simulink model "lab3_real_integrator"  (R2015a)
settings: Solver=ode3  StartTime=0.0  StopTime=30  RelTol=1e-3
values from neighbouring files (symbols this model uses):
  Ke = -4.2046    [controller_design.m]    (also in controller_test.m)
  Kp = 34.0683    [controller_design.m]    (also in controller_test.m)
  Nbar = Nu+K*Nx    [controller_design.m]    (also in controller_test.m)
  sampling_time = 1/50    (= 0.02)    [controller_design.m]    (also in controller_test.m)
undefined symbols (not defined in the file or in its folder): A, B, C, K, M, MIO, National_Instruments, PCI
libraries: sldrtlib x2
settings Model: SimulationMode=external  ExtModeTrigDuration=200000  Creator=alunos  LastModifiedBy=alunos
settings DataIOCC: LimitDataPoints=off
settings HardwareCC: ProdBitPerPointer=64  ProdLargestAtomicFloat=Float  ProdIntDivRoundTo=Zero  ProdEndianess=LittleEndian  ProdHWDeviceType=Specified  TargetIntDivRoundTo=Zero  TargetEndianess=LittleEndian  TargetHWDeviceType=Intel->x86/Pentium
settings RTWCC: SystemTargetFile=rtwin.tlc  TemplateMakefile=rtwin.tmf  Description=Simulink Desktop Real-Time  RTWCompilerOptimization=on
settings CodeAppCC: MaxIdLength=95
settings RTWinTargetCC: TargetPreCompLibLocation=C:\Program Files\MATLAB\R2017a\toolbox\sldrt\lib\win64  ExtModeMexFile=sldrtext

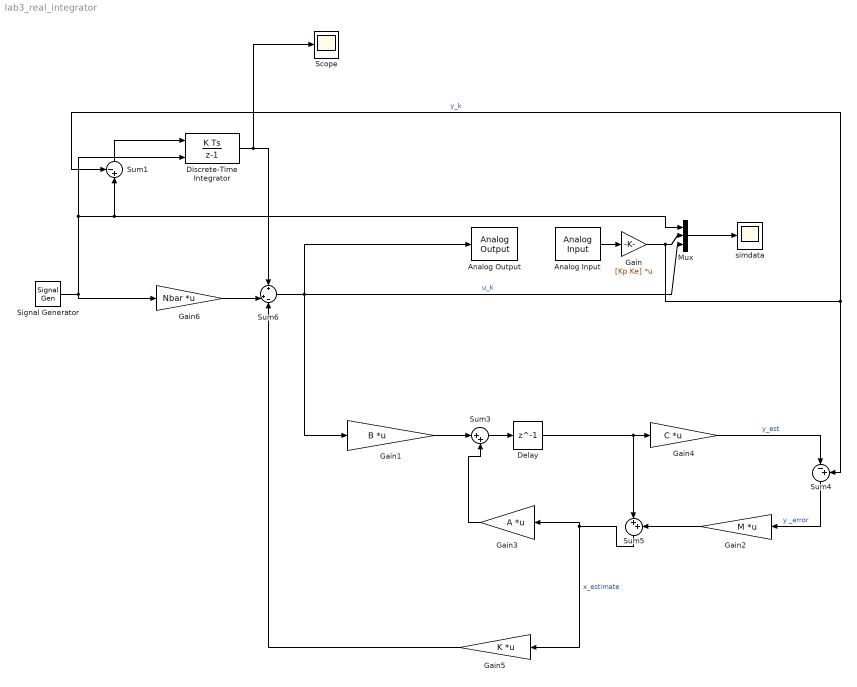
== system lab3_real_integrator ==
  Analog Input : sldrtlib/Analog Input  SampleTime=sampling_time  MaxMissedTicks=10  ShowMissedTicks=off  YieldWhenWaiting=off  DrvName=National_Instruments/PCI-MIO-16E-4  DrvAddress=4294967295  DrvOptions=[0 0 0 0 0 0]  Channels=[1 2]  RangeMode=1  VoltRange=1  DataType=1
      settings: AttributesFormatString=National Instruments\nPCI-MIO-16E-4 [auto]
  Analog Output : sldrtlib/Analog Output  SampleTime=sampling_time  MaxMissedTicks=10  ShowMissedTicks=off  YieldWhenWaiting=off  DrvName=National_Instruments/PCI-MIO-16E-4  DrvAddress=4294967295  DrvOptions=[0 0 0 0 0 0]  Channels=1  RangeMode=1  VoltRange=1  InitialValue=0  FinalValue=0
      settings: AttributesFormatString=National Instruments\nPCI-MIO-16E-4 [auto]
  Delay : Delay  DelayLength=1
  Discrete-Time Integrator : DiscreteIntegrator  gainval=0.15  ExternalReset=either  InitialConditionSetting=State (most efficient)  SampleTime=0.02  LimitOutput=on  UpperSaturationLimit=0.42  LowerSaturationLimit=-0.46
  Gain : Gain  Gain=[Kp Ke]  Multiplication=Matrix(K*u)
  Gain1 : Gain  Gain=B  Multiplication=Matrix(K*u)
  Gain2 : Gain  Gain=M  Multiplication=Matrix(K*u)
  Gain3 : Gain  Gain=A  Multiplication=Matrix(K*u)
  Gain4 : Gain  Gain=C  Multiplication=Matrix(K*u)
  Gain5 : Gain  Gain=K  Multiplication=Matrix(K*u)
  Gain6 : Gain  Gain=Nbar  Multiplication=Matrix(K*u)
  Mux : Mux  Inputs=3
  Scope : Scope
      settings: TickLabels=on  SaveName=integratordata  SampleInput=on  SampleTime=0.02
  Signal Generator : SignalGenerator  WaveForm=square  Amplitude=30
  Sum1 : Sum  Inputs=-+|
  Sum3 : Sum  Inputs=|++
  Sum4 : Sum  Inputs=|-+
  Sum5 : Sum  Inputs=|++
  Sum6 : Sum  Inputs=+|+-
  simdata : Scope
      settings: TickLabels=on  YMin=-40  YMax=35  SaveName=simdata  SampleInput=on  SampleTime=sampling_time_scope
  wires:
  Mux/1 -> simdata/1
  Gain1/1 -> Sum3/1
  Sum3/1 -> Delay/1
  Delay/1 -> Gain4/1, Sum5/1
  Sum4/1 -> Gain2/1  "y _error"
  Gain2/1 -> Sum5/2
  Gain3/1 -> Sum3/2
  Gain/1 -> Mux/2, Sum4/2, Sum1/1  "y_k"
  Sum5/1 -> Gain3/1, Gain5/1  "x_estimate"
  Gain4/1 -> Sum4/1  "y_est"
  Sum6/1 -> Mux/3, Gain1/1, Analog Output/1  "u_k"
  Gain5/1 -> Sum6/3
  Signal Generator/1 -> Discrete-Time Integrator/2, Sum1/2, Mux/1, Gain6/1
  Analog Input/1 -> Gain/1
  Gain6/1 -> Sum6/2
  Sum1/1 -> Discrete-Time Integrator/1
  Discrete-Time Integrator/1 -> Scope/1, Sum6/1
